simulink model "No_2_Simulink"  (R2023b)
settings: Solver=VariableStepAuto  StartTime=0.0  StopTime=20  RelTol=1e-3
values from neighbouring files (symbols this model uses):
  G1_den = [1 0 0]    [No_1.m]    (also in No_2.m)
  G1_num = [1]    [No_1.m]    (also in No_2.m)
  G2_den = [1 1]    [No_1.m]    (also in No_2.m)
  G2_num = [1]    [No_1.m]    (also in No_2.m)
  G3_den = [1 0]    [No_1.m]    (also in No_2.m)
  G3_num = [1]    [No_1.m]    (also in No_2.m)
  G4_den = [2 0]    [No_2.m]
  G4_num = [1]    [No_2.m]
  H1_den = [1 0]    [No_1.m]    (also in No_2.m)
  H1_num = [1]    [No_1.m]    (also in No_2.m)
  H2_den = [1 -1]    [No_1.m]    (also in No_2.m)
  H2_num = [1]    [No_1.m]    (also in No_2.m)
  H3_den = [1 -2]    [No_1.m]    (also in No_2.m)
  H3_num = [1]    [No_1.m]    (also in No_2.m)
  TF3_den = conv(G2_den,G2H2_den_sum)    [No_1.m]    (also in No_2.m = conv(G1G2G3G4_den,G1G2G3G4H1_den_sum))
  TF3_num = conv(G2_num,G2H2_den)    [No_1.m]    (also in No_2.m = conv(TF2_num,G1G2G3G4H1_den))
settings Model: Creator=Corinne  LastModifiedBy=Corinne

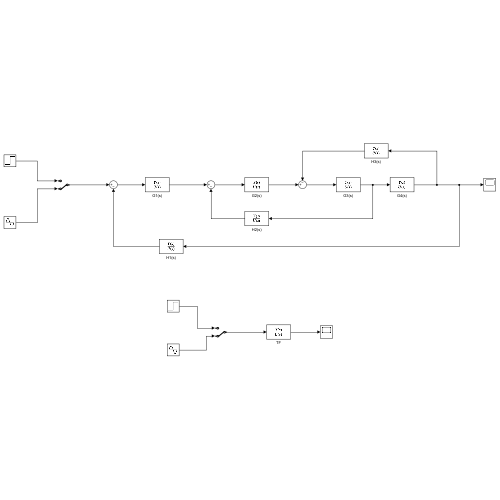
[thumbnail: Simulink's stored preview of the top-level diagram]
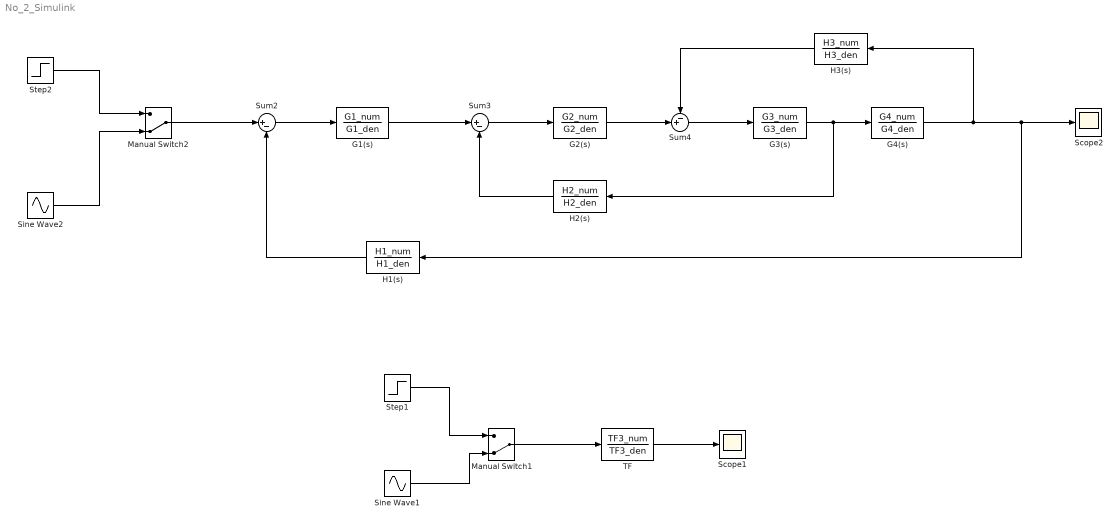
== system No_2_Simulink ==
  G1(s) : TransferFcn  Numerator=G1_num  Denominator=G1_den
  G2(s) : TransferFcn  Numerator=G2_num  Denominator=G2_den
  G3(s) : TransferFcn  Numerator=G3_num  Denominator=G3_den
  G4(s) : TransferFcn  Numerator=G4_num  Denominator=G4_den
  H1(s) : TransferFcn  Numerator=H1_num  Denominator=H1_den
  H2(s) : TransferFcn  Numerator=H2_num  Denominator=H2_den
  H3(s) : TransferFcn  Numerator=H3_num  Denominator=H3_den
  Manual Switch1 : ManualSwitch  CurrentSetting=0
  Manual Switch2 : ManualSwitch  CurrentSetting=0
  Scope1 : Scope
  Scope2 : Scope
  Sine Wave1 : Sin  SampleTime=0
  Sine Wave2 : Sin  SampleTime=0
  Step1 : Step  SampleTime=0
  Step2 : Step  SampleTime=0
  Sum2 : Sum  Inputs=|+-
  Sum3 : Sum  Inputs=|+-
  Sum4 : Sum  Inputs=-+|
  TF : TransferFcn  Numerator=TF3_num  Denominator=TF3_den
  wires:
  Step1/1 -> Manual Switch1/1
  Sine Wave1/1 -> Manual Switch1/2
  Manual Switch1/1 -> TF/1
  TF/1 -> Scope1/1
  Sine Wave2/1 -> Manual Switch2/2
  Manual Switch2/1 -> Sum2/1
  Step2/1 -> Manual Switch2/1
  H1(s)/1 -> Sum2/2
  H2(s)/1 -> Sum3/2
  G1(s)/1 -> Sum3/1
  Sum2/1 -> G1(s)/1
  Sum3/1 -> G2(s)/1
  G2(s)/1 -> Sum4/2
  Sum4/1 -> G3(s)/1
  G3(s)/1 -> H2(s)/1, G4(s)/1
  H3(s)/1 -> Sum4/1
  G4(s)/1 -> H3(s)/1, H1(s)/1, Scope2/1
